simulink subsystem "TrajectoryGenerator"  (R2021a)
settings: Solver=VariableStepAuto  StartTime=0.0  StopTime=10.0  RelTol=1e-3
settings Model: Creator=Sirius  LastModifiedBy=Sirius

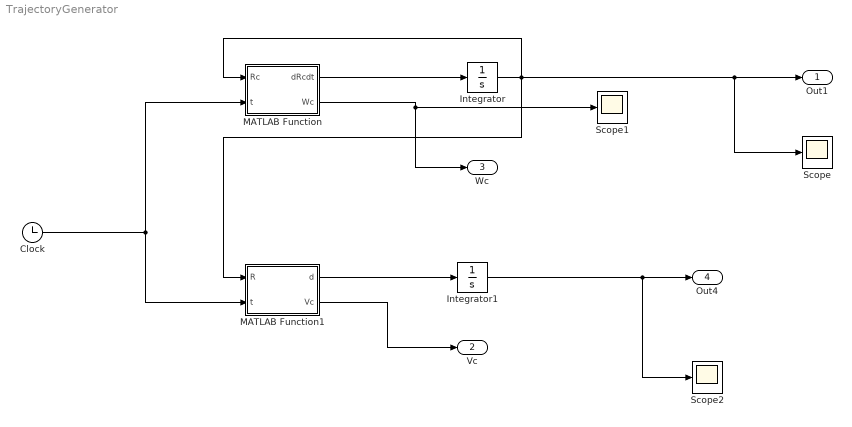
== system TrajectoryGenerator ==
  Clock : Clock
  Integrator : Integrator
  Integrator1 : Integrator
  MATLAB Function : MATLAB Function  TreatAsAtomicUnit=on
  MATLAB Function1 : MATLAB Function  TreatAsAtomicUnit=on
  Scope : Scope
  Scope1 : Scope
  Scope2 : Scope
  Out1 : Outport
  Vc : Outport  Port=2
  Wc : Outport  Port=3
  Out4 : Outport  Port=4
  wires:
  MATLAB Function/2(Wc) -> Wc/1, Scope1/1
  Integrator/1 -> MATLAB Function1/1(R), MATLAB Function/1(Rc), Scope/1, Out1/1
  MATLAB Function/1(dRcdt) -> Integrator/1
  Clock/1 -> MATLAB Function/2(t), MATLAB Function1/2(t)
  Integrator1/1 -> Scope2/1, Out4/1
  MATLAB Function1/1(d) -> Integrator1/1
  MATLAB Function1/2(Vc) -> Vc/1

== matlab function TrajectoryGenerator/MATLAB Function ==
  data: Rc input; dRcdt output; t input; Wc output
function [dRcdt,Wc] =R(Rc,t)

Wc=[0;0;0];
if((t>=19.5)&&(t<=20.5))
    Wc=[0;0;pi/2];
end
if((t>=39.5)&&(t<=40.5))
    Wc=[0;0;pi/2];
end
if((t>=59.5)&&(t<=60.5))
    Wc=[0;0;pi/2];
end
dRcdt=R*Skew(Wc)
end

== matlab function TrajectoryGenerator/MATLAB Function1 ==
  data: R input; d output; t input; Vc output
function [d,Vc] = P(R,t)
Vc=[0.5;0;0]
dPdt=R*Vc;

end
